simulink model "hw2"  (Simulink 8.5)
settings: Solver=ode45  StartTime=0.0  StopTime=150  RelTol=1e-3
values from neighbouring files (symbols this model uses):
  bi = 1    [macro.m]
undefined symbols (not defined in the file or in its folder): K
settings Model: Creator=kallej  LastModifiedBy=enriquejcobo  ExtModeTrigMode=oneshot  ExtModeArmWhenConnect=off
settings DataIOCC: LimitDataPoints=off
settings OptimizationCC: BlockReduction=off  BooleanDataType=off  ExpressionDepthLimit=128
settings DebuggingCC: SaveWithParameterizedLinksMsg=none  SignalResolutionControl=TryResolveAllWithWarning  MultiTaskDSMMsg=warning  MultiTaskCondExecSysMsg=none  FcnCallInpInsideContextMsg=EnableAllAsError  StateNameClashWarn=none
settings HardwareCC: TargetUnknown=on

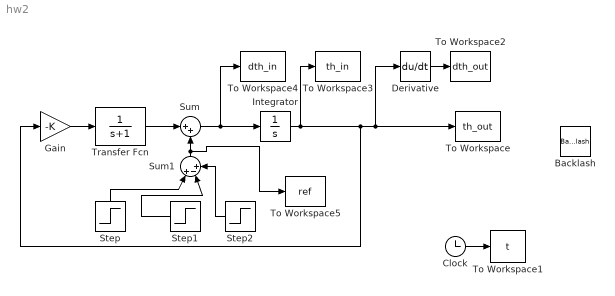
== system hw2 ==
  Backlash : Backlash
  Clock : Clock
  Derivative : Derivative
  Gain : Gain  Gain=-K  SaturateOnIntegerOverflow=on  OutDataTypeStr=Inherit: Same as input  ParamDataTypeStr=Inherit: Same as input
  Integrator : Integrator
  Step : Step  SampleTime=0
  Step1 : Step  Time=2  After=1+bi  SampleTime=0
  Step2 : Step  Time=3  After=bi  SampleTime=0
  Sum : Sum  Inputs=|++  SaturateOnIntegerOverflow=on  InputSameDT=on  OutDataTypeStr=Inherit: Same as first input
  Sum1 : Sum  Inputs=|+-+  SaturateOnIntegerOverflow=on  InputSameDT=on  OutDataTypeStr=Inherit: Same as first input
  To Workspace : ToWorkspace  VariableName=th_out  SampleTime=-1
  To Workspace1 : ToWorkspace  VariableName=t  SampleTime=-1
  To Workspace2 : ToWorkspace  VariableName=dth_out  SampleTime=-1
  To Workspace3 : ToWorkspace  VariableName=th_in  SampleTime=-1
  To Workspace4 : ToWorkspace  VariableName=dth_in  SampleTime=-1
  To Workspace5 : ToWorkspace  VariableName=ref  SampleTime=-1
  Transfer Fcn : TransferFcn  Denominator=[1 1]
  wires:
  Derivative/1 -> To Workspace2/1
  Transfer Fcn/1 -> Sum/1
  Gain/1 -> Transfer Fcn/1
  Clock/1 -> To Workspace1/1
  Sum/1 -> To Workspace4/1, Integrator/1
  Step/1 -> Sum1/1
  Step1/1 -> Sum1/2
  Sum1/1 -> To Workspace5/1, Sum/2
  Step2/1 -> Sum1/3
  Integrator/1 -> Gain/1, Derivative/1, To Workspace/1, To Workspace3/1
